simulink model "Parameters_supp"  (R2022b)
settings: Solver=ode4  StartTime=0.0  StopTime=20  FixedStep=0.0001  RelTol=1e-3
values from neighbouring files (symbols this model uses):
  Ap = 4.91e-4    (= 0.000491)    [Parameters_supp(1).m]
  m1f = m    (= 6)    [Parameters_supp(1).m]
  ps = 4e6    (= 4000000)    [Parameters_supp(1).m]
  theta1 = k/m    (= 166.666666667)    [Parameters_supp(1).m]
  theta2 = b/m    (= 8.33333333333)    [Parameters_supp(1).m]
  theta3 = 1/m    (= 0.166666666667)    [Parameters_supp(1).m]
  theta4 = (4*beta_e*Ap^2)/Vt    (= 7723418.7643)    [Parameters_supp(1).m]
  theta5 = (4*beta_e*Ap*Ctl)/Vt    (= 0.393249427918)    [Parameters_supp(1).m]
  theta6 = (4*beta_e*Cd*w*Ksv*Ap)/(Vt*(rho)^(1/2))    (= 4014.13120392)    [Parameters_supp(1).m]
undefined symbols (not defined in the file or in its folder): sgn
libraries: dsparch4 x6
settings Model: Creator=maxinbao  LastModifiedBy=Administrator
settings SolverCC: AlgebraicLoopSolver=TrustRegion
settings DebuggingCC: UnconnectedInputMsg=warning  UnconnectedOutputMsg=warning  UnconnectedLineMsg=warning  SFMachineParentedDataDiag=warning  ArithmeticOperatorsInVariantConditions=warning
settings ModelReferenceCC: EnableRefExpFcnMdlSchedulingChecks=on
settings SFSimCC: CustomCodeUndefinedFunction=UseInterfaceOnly
settings CodeAppCC: StateflowObjectComments=on

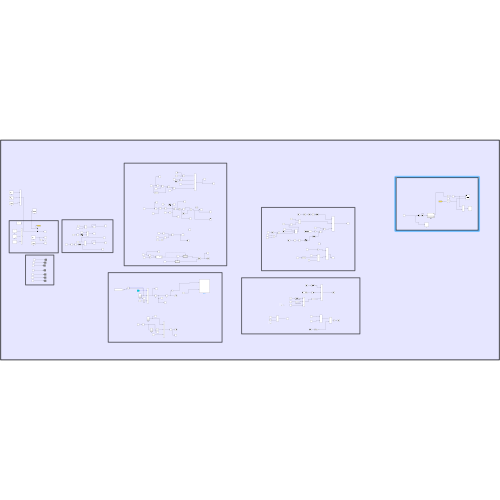
[thumbnail: Simulink's stored preview of the top-level diagram]
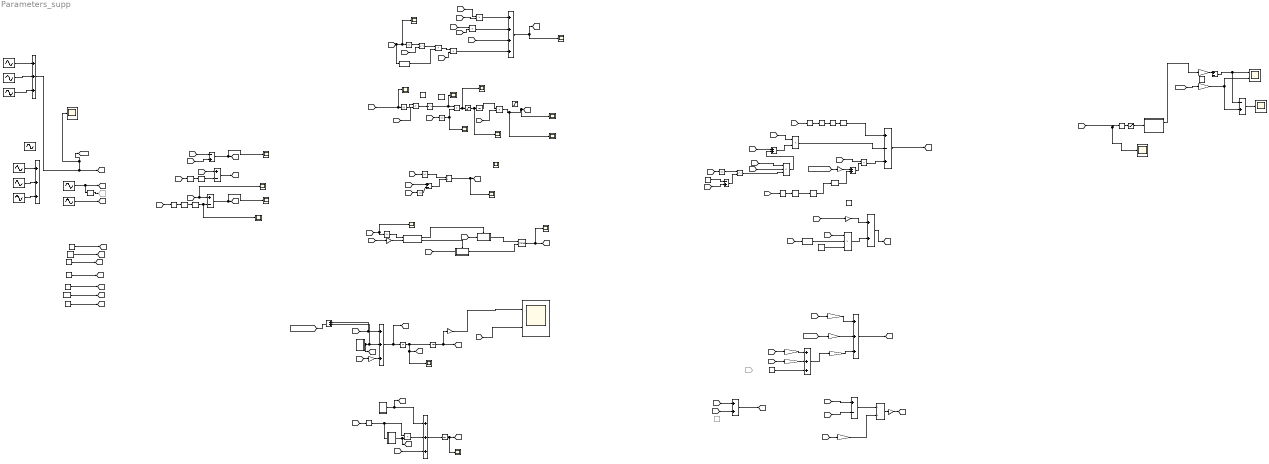
== system Parameters_supp ==
  1/m1 : Gain  Gain=theta3
  4*beta_e*Ap/Vt : Gain  Gain=-theta4
  4*beta_e*Ctl/Vt : Gain  Gain=-theta5
  Abs{,1..6} (7 alike) : Abs  SaturateOnIntegerOverflow=off
  Add{,1,8,11,16} (5 alike) : Sum
  Add{2..3,9..10,12..13} (6 alike) : Sum  Inputs=+++
  Add14 : Sum  Inputs=++++
  Add15 : Sum  Inputs=-+
  Add4 : Sum  Inputs=-+
  Add5 : Sum  Inputs=-+
  Add6 : Sum  Inputs=+-
  Add7 : Sum  Inputs=+-
  Analog Filter Design{1..6} (6 alike) : dsparch4/Analog Filter Design  method=Butterworth  filttype=Lowpass  N=8  Wlo=30  Whi=80  Rp=2  Rs=40
  Constant : Constant  Value=0.1
  Constant1 : Constant  Value=0.000001
  Constant10 : Constant  Value=5
  Constant11 : Constant  Commented=on  Value=0
  Constant12 : Constant  Value=55000
  Constant13 : Constant
  Constant2 : Constant  Value=0.3
  Constant3 : Constant  Value=50
  Constant4 : Constant  Value=200
  Constant5 : Constant  Value=0
  Constant6 : Constant  Value=2.6
  Constant7 : Constant  Value=1.55
  Constant8 : Constant  Value=-1
  Constant9 : Constant  Value=0
  Derivative{1..3,7..8,10..13} (9 alike) : Derivative
  Divide : Product  Inputs=*/
  Divide4 : Product  Inputs=*/
  EHS1 : Subsystem
  Fcn : Fcn  Expr=sgn(u(1))
  Fcn3 : Fcn  Expr=sgn(u(1))
  From56 : From  Commented=on  GotoTag=DELTA3  TagVisibility=global
  Gain : Gain  Gain=0.5
  Gain1 : Gain  Gain=-theta1
  Gain2 : Gain  Gain=-theta2
  Gain3 : Gain  Gain=theta3
  Gain4 : Gain  Gain=theta3
  Gain5 : Gain
  Gain6 : Gain
  Gain7 : Gain  Gain=-1
  Gain8 : Gain  Gain=-20
  Goto14 : Goto  Commented=on  GotoTag=delta  TagVisibility=global
  If : If  NumInputs=2  IfExpression=u1 >= u2
  If Action Subsystem : Subsystem  TreatAsAtomicUnit=on
  If Action Subsystem1 : Subsystem  TreatAsAtomicUnit=on
  Integrator : Integrator
  Math Function : Math  Operator=pow  SignedPower=on
  Math Function1 : Math  SignedPower=on
  Math Function2 : Math  Operator=pow  SignedPower=on
  Memory1 : Memory
  Memory9 : Memory
  Merge : Merge
  Product{,3..8,11,13} (9 alike) : Product
  Product10 : Product  Inputs=3
  Product2 : Product  RndMeth=Zero
  Product9 : Product  Inputs=3
  Saturation : Saturate  UpperLimit=10380  LowerLimit=-10380
  Saturation1 : Saturate  UpperLimit=0.5e10  LowerLimit=-0.5e10
  Scope{,2..19} (19 alike) : Scope
  Scope1 : Scope  NumInputPorts=2
  Subtract : Sum  Inputs=+-
  Subtract2 : Sum  Inputs=+-
  Subtract3 : Sum  Inputs=+-+
  e_x : Scope
  fi2(t)1 : Subsystem
  fi3(t)1 : Subsystem
  gi3(t)1 : Subsystem
  ob_u : Sum  Inputs=+-
  u : Gain  Gain=1000
  u3 : Scope
  u_three2 : Saturate  UpperLimit=2  LowerLimit=-2
  x1 : Integrator
  x2 : Integrator  InitialCondition=0.02
  x3 : Integrator
  xd : Sin  Amplitude=0.02  Frequency=pi  SampleTime=0
  xd1 : Sin  Amplitude=10  Frequency=pi  SampleTime=0
  xd2 : Sin  Amplitude=2000  Frequency=pi  SampleTime=0
  xd3 : Sin  Amplitude=0.05/2  Frequency=pi  SampleTime=0
  xd4 : Sin  Amplitude=0.04/3  Frequency=pi/3  SampleTime=0
  xd5 : Sin  Amplitude=0.05/2  Frequency=pi/2  SampleTime=0
  xd6 : Sin  Amplitude=0.04/3  Frequency=pi  SampleTime=0
  xd7 : Sin  Amplitude=0.04/3  Frequency=pi/3  SampleTime=0
  xd8 : Sin  Amplitude=0.04/3  Frequency=pi/4  SampleTime=0
  yd : Gain  Gain=1000
  yd1 : Scope
  位置跟踪效果对比 : Scope  NumInputPorts=2
  tag scope: DELTA2=global, DELTA3=global, a=global, alpha=global, dde=global, de=global, dx2=global, dx2WithoutDELTA=global, e=global, epsilon=global, eta=global, f2_bf=global, f3_bf=global, g3_bf=global, gama=global, k_hat1=global, k_hat2=global, k_hat=global, lamda0=global, lamda1=global, lf3h=global, s=global, u0=global, v1=global, v2=global, v=global, x1_bf=global, x2_bf=global, x3_bf=global, xd=global, yd=global
  wires:
  Add7/1 -> Scope14/1, [dde]
  [v2] -> Add11/2
  xd5/1 -> Add10/3
  [epsilon] -> Subtract/1
  Math Function1/1 -> Scope6/1, Product4/1
  xd4/1 -> Add10/2
  Analog Filter Design5/1 -> Subtract3/1
  xd3/1 -> Add10/1
  Constant3/1 -> [gama]
  Divide4/1 -> Gain5/1
  Derivative12/1 -> Analog Filter Design5/1
  [s] -> Scope10/1, Abs2/1
  Product2/1 -> Add3/2
  [lf3h] -> Subtract2/2
  [x1] -> Add4/2
  Product5/1 -> Scope8/1, [k_hat1], Scope12/1
  Add12/1 -> Gain3/1
  Derivative7/1 -> Goto14/1
  Saturation1/1 -> Scope5/1, Integrator/1
  Derivative11/1 -> Derivative13/1
  If Action Subsystem/1(Out1) -> Merge/1
  [DELTA3] -> Add3/3
  [s] -> Abs3/1
  fi2(t)1/1(Out1) -> Add/2, Add2/2, [f2_bf]
  Gain1/1 -> Add13/1
  x2/1 -> Scope19/1, [x2_bf], x1/1
  Add11/1 -> [v]
  Analog Filter Design4/1 -> Add6/2
  [x2] -> 4*beta_e*Ap/Vt/1
  Constant8/1 -> Product10/3
  Constant/1 -> [epsilon]
  Abs4/1 -> Divide/1
  1/m1/1 -> Add2/3
  [xd] -> Derivative3/1
  Add6/1 -> [de]
  [dx2] -> Scope15/1, Add7/1
  If Action Subsystem1/1(Out1) -> Merge/2
  Product4/1 -> Scope13/1, Saturation1/1
  [e] -> Scope17/1, Abs/1, Fcn/1
  Integrator/1 -> Product5/1
  Derivative3/1 -> Analog Filter Design4/1
  [a] -> Math Function/2
  [xd] -> Add4/1
  [g3_bf] -> Gain4/1
  Fcn3/1 -> Product10/2
  Constant1/1 -> [eta]
  Derivative2/1 -> Derivative1/1
  If/2 -> If Action Subsystem1/Action
  [k_hat] -> Product10/1
  Add4/1 -> Scope11/1, [e]
  Analog Filter Design1/1 -> Scope16/1, Add7/2
  [x2] -> Gain1/1
  Constant2/1 -> [alpha]
  [epsilon] -> Gain/1
  Constant9/1 -> Add12/3
  [eta] -> Product5/2
  [s] -> Abs5/1
  Product6/1 -> Add14/2
  Gain5/1 -> [u0]
  [v] -> Subtract2/1
  Constant4/1 -> [lamda1]
  Gain/1 -> If/2
  [k_hat1] -> If Action Subsystem/1(In1)
  Abs/1 -> Math Function/1
  [s] -> Fcn3/1
  Gain4/1 -> Divide4/2
  [xd] -> Scope1/2
  [k_hat2] -> If Action Subsystem1/1(In1)
  [alpha] -> Product3/2
  [DELTA2] -> Add/1, Add2/1
  x1/1 -> Gain6/1, [x1_bf]
  [v1] -> Add11/1
  [xd] -> Derivative11/1
  Add3/1 -> x3/1
  [s] -> Scope4/1, Abs1/1
  Derivative1/1 -> Analog Filter Design1/1
  Merge/1 -> Scope2/1, [k_hat]
  [s] -> Abs4/1
  [xd] -> Derivative2/1
  gi3(t)1/1(Out1) -> [g3_bf], Product2/2
  [lamda0] -> Product11/1
  Subtract3/1 -> [v1]
  Abs1/1 -> If/1
  Add14/1 -> [s], Scope/1
  x3/1 -> Scope3/1, [x3_bf]
  4*beta_e*Ap/Vt/1 -> Add12/1
  Abs2/1 -> Product3/1
  Product8/1 -> Subtract3/2
  [lamda1] -> Product6/2
  Math Function/1 -> Product/1
  Abs5/1 -> Subtract/2
  Add2/1 -> [dx2], x2/1
  Fcn/1 -> Product/2
  xd1/1 -> Derivative7/1, [DELTA2]
  Product11/1 -> Add14/1
  Subtract/1 -> Divide/2
  [x2] -> Add6/1
  Abs3/1 -> Scope7/1, Product4/2
  Constant12/1 -> [lamda0]
  Add13/1 -> [lf3h]
  [dx2WithoutDELTA] -> Gain2/1
  Gain2/1 -> Add13/2
  [x3] -> 1/m1/1
  xd2/1 -> [DELTA3]
  Product3/1 -> Math Function1/1
  Gain3/1 -> Add13/3
  If/1 -> If Action Subsystem/Action
  Subtract2/1 -> Divide4/1
  Memory1/1 -> gi3(t)1/1(In1), Product2/1
  Add/1 -> [dx2WithoutDELTA]
  Derivative13/1 -> Derivative12/1
  [x3] -> 4*beta_e*Ctl/Vt/1
  Gain6/1 -> Scope1/1
  Divide/1 -> Scope9/1, [k_hat2]
  fi3(t)1/1(Out1) -> Add3/1, [f3_bf]
  [de] -> Product6/1
  [u0] -> Memory1/1
  4*beta_e*Ctl/Vt/1 -> Add12/2
  [e] -> Product11/2
  [dde] -> Add14/3
  Constant7/1 -> [a]
  Product/1 -> Product7/1
  [gama] -> Product7/2
  [de] -> Product8/1
  [lamda0] -> Add8/1
  [gama] -> Product9/1
  [a] -> Product9/2
  Add15/1 -> Math Function2/2
  [a] -> Add15/2
  Constant13/1 -> Add15/1
  [e] -> Abs6/1
  Abs6/1 -> Math Function2/1
  Math Function2/1 -> Product9/3
  Product9/1 -> Add8/2
  Add8/1 -> Product8/2
  [lamda1] -> Product13/1
  Add16/1 -> Product13/2
  Product13/1 -> Subtract3/3
  [dx2WithoutDELTA] -> Gain7/1
  Gain7/1 -> Add16/1
  [xd] -> Derivative8/1
  Derivative8/1 -> Derivative10/1
  Derivative10/1 -> Analog Filter Design2/1
  Analog Filter Design6/1 -> Add16/2
  Analog Filter Design2/1 -> Analog Filter Design6/1
  Add1/1 -> [v2]
  Product10/1 -> Add1/2
  [s] -> Gain8/1
  Gain8/1 -> Add1/1
  ob_u/1 -> Add5/1, 位置跟踪效果对比/1
  Add5/1 -> e_x/1
  yd/1 -> 位置跟踪效果对比/2, Add5/2
  [yd] -> yd/1
  EHS1/1(x11) -> u/1
  u/1 -> ob_u/1
  Memory9/1 -> u_three2/1
  [u0] -> u3/1, Memory9/1
  u_three2/1 -> EHS1/1(u)
  xd6/1 -> Add9/1
  xd7/1 -> Add9/2
  xd8/1 -> Add9/3
  Add9/1 -> yd1/1, [yd], [xd]
  Product7/1 -> Add14/4

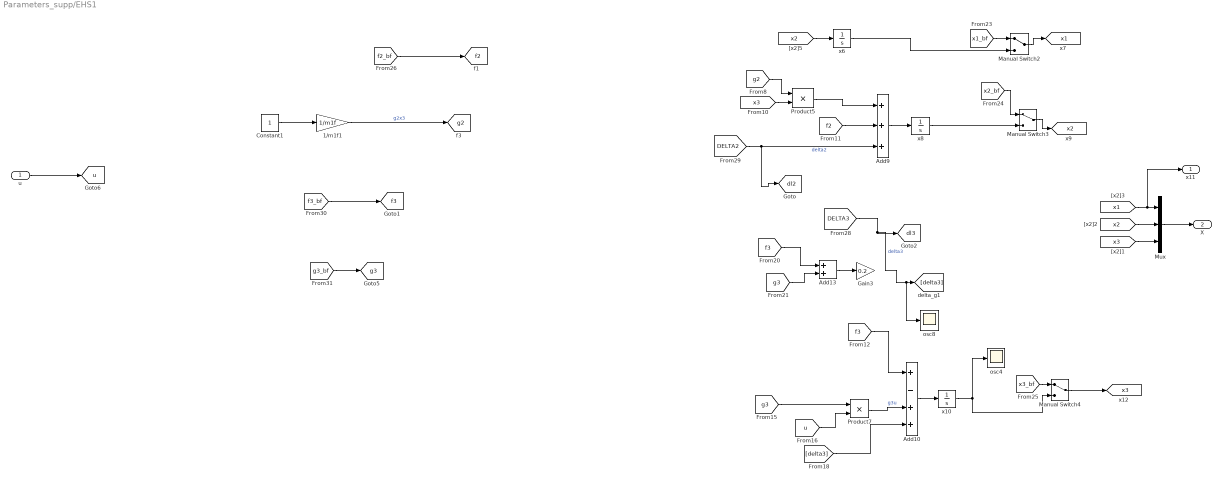
== system Parameters_supp/EHS1 ==
  u : Inport
  1/m1f1 : Gain  Gain=1/m1f
  Add10 : Sum  Inputs=+-++
  Add13 : Sum
  Add9 : Sum  Inputs=+++
  Constant1 : Constant
  Gain3 : Gain  Gain=0.2
  Manual Switch2 : ManualSwitch
  Manual Switch3 : ManualSwitch
  Manual Switch4 : ManualSwitch
  Mux : Mux  Inputs=3
  Product5 : Product  RndMeth=Zero
  Product7 : Product
  osc4 : Scope
  osc8 : Scope
  x10 : Integrator  UpperSaturationLimit=40e5  LowerSaturationLimit=-40e5
  x6 : Integrator
  x8 : Integrator
  x11 : Outport
  X : Outport  Port=2
  tag scope: dl2=global, dl3=global, f2=global, f3=global, g2=global, g3=global, u=global, x1=global, x2=global, x3=global
  wires:
  [x2] -> Mux/2
  [x3] -> Mux/3
  Mux/1 -> X/1
  [x2] -> x6/1
  Constant1/1 -> 1/m1f1/1
  1/m1f1/1 -> [g2]  "g2x3"
  Add9/1 -> x8/1
  Product5/1 -> Add9/1
  [x3] -> Product5/2
  [g2] -> Product5/1
  [f2] -> Add9/2
  [DELTA2] -> [dl2], Add9/3  "delta2"
  Add10/1 -> x10/1
  [f3] -> Add10/1
  Product7/1 -> Add10/3  "g3u"
  [u] -> Product7/2
  [g3] -> Product7/1
  [f3] -> Add13/1
  [g3] -> Add13/2
  Add13/1 -> Gain3/1
  [DELTA3] -> osc8/1, [delta3], [dl3]  "delta3"
  [delta3] -> Add10/4
  [x1] -> x11/1, Mux/1
  u/1 -> [u]
  x6/1 -> Manual Switch2/2
  x8/1 -> Manual Switch3/2
  x10/1 -> Manual Switch4/2, osc4/1
  Manual Switch2/1 -> [x1]
  [x1_bf] -> Manual Switch2/1
  [x2_bf] -> Manual Switch3/1
  Manual Switch3/1 -> [x2]
  [x3_bf] -> Manual Switch4/1
  Manual Switch4/1 -> [x3]
  [f2_bf] -> [f2]
  [f3_bf] -> [f3]
  [g3_bf] -> [g3]

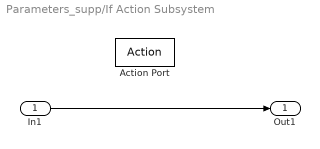
== system Parameters_supp/If Action Subsystem ==
  In1 : Inport
  Action Port : ActionPort  ActionPortLabel=if(u1 >= u2)
  Out1 : Outport
  wires:
  In1/1 -> Out1/1

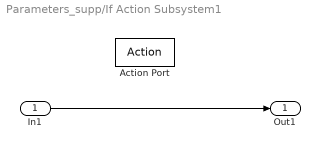
== system Parameters_supp/If Action Subsystem1 ==
  In1 : Inport
  Action Port : ActionPort  ActionPortLabel=else
  Out1 : Outport
  wires:
  In1/1 -> Out1/1

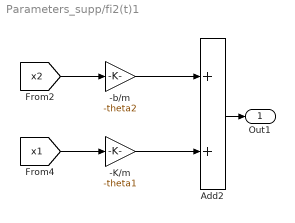
== system Parameters_supp/fi2(t)1 ==
  -K/m : Gain  Gain=-theta1
  -b/m : Gain  Gain=-theta2
  Add2 : Sum
  Out1 : Outport
  wires:
  [x1] -> -K/m/1
  -K/m/1 -> Add2/2
  -b/m/1 -> Add2/1
  Add2/1 -> Out1/1
  [x2] -> -b/m/1

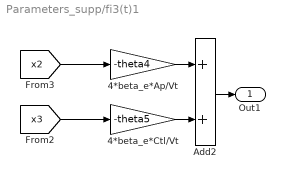
== system Parameters_supp/fi3(t)1 ==
  4*beta_e*Ap/Vt : Gain  Gain=-theta4
  4*beta_e*Ctl/Vt : Gain  Gain=-theta5
  Add2 : Sum
  Out1 : Outport
  wires:
  [x2] -> 4*beta_e*Ap/Vt/1
  Add2/1 -> Out1/1
  4*beta_e*Ctl/Vt/1 -> Add2/2
  [x3] -> 4*beta_e*Ctl/Vt/1
  4*beta_e*Ap/Vt/1 -> Add2/1

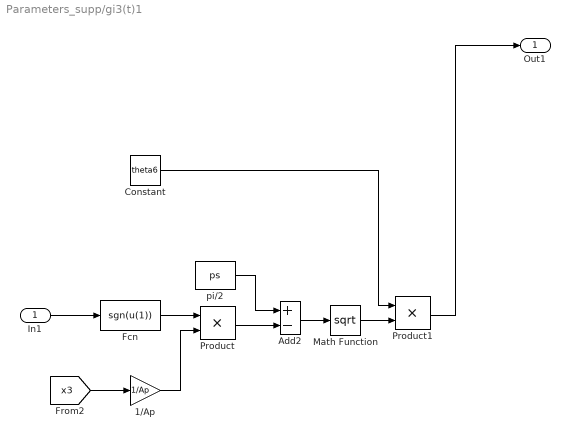
== system Parameters_supp/gi3(t)1 ==
  In1 : Inport
  "1/Ap " : Gain  Gain=1/Ap
  Add2 : Sum  Inputs=+-
  Constant : Constant  Value=theta6
  Fcn : Fcn  Expr=sgn(u(1))
  Math Function : Math  Operator=sqrt  SignedPower=on
  Product : Product  RndMeth=Zero
  Product1 : Product  RndMeth=Zero
  pi/2 : Constant  Value=ps  VectorParams1D=off
  Out1 : Outport
  wires:
  [x3] -> "1/Ap "/1
  "1/Ap "/1 -> Product/2
  Add2/1 -> Math Function/1
  Fcn/1 -> Product/1
  Constant/1 -> Product1/1
  Product/1 -> Add2/2
  Math Function/1 -> Product1/2
  Product1/1 -> Out1/1
  pi/2/1 -> Add2/1
  In1/1 -> Fcn/1
